simulink model "float_mch_LocalMaxima_HardThreshold"  (R2020a)
settings: Solver=VariableStepAuto  StartTime=0.0  StopTime=10  RelTol=1e-3
model workspace (MAT data in the model file):
  a = 0
values from neighbouring files (symbols this model uses):
  fs = 30000    [float_mch_run_LocalMaxima_AdaptiveThreshold.m]    (also in float_mch_run_LocalMaxima_HardThreshold.m)
libraries: dspfdesign x2, dspswit3 x1, simulink x1
settings Model: SimulationMode=accelerator  Creator=sbuccelli  LastModifiedBy=diflo

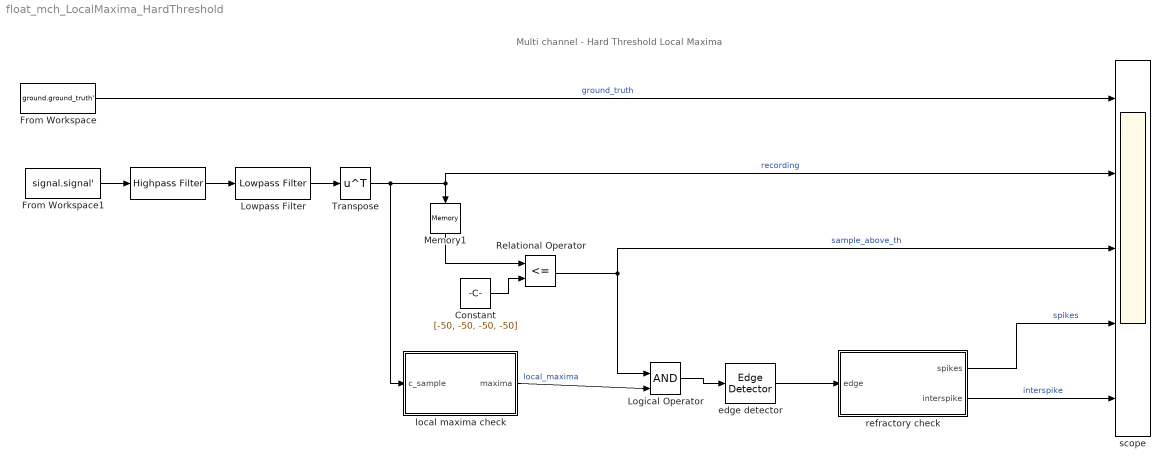
== system float_mch_LocalMaxima_HardThreshold ==
  note: Multi channel - Hard Threshold Local Maxima
  " " : dspfdesign/Highpass Filter  FilterType=IIR  DesignForMinimumOrder=on  FilterOrder=50  StopbandFrequency=1  PassbandFrequency=300  StopbandAttenuation=80  PassbandRipple=0.1  InheritSampleRate=off  SampleRate=30000  SimulateUsing=Interpreted execution  roundingMode=Floor  coeffsDataTypeStr=fixdt(1,16)
  Constant : Constant  Value=[-50, -50, -50, -50]
  From Workspace : FromWorkspace  VariableName=ground.ground_truth'  SampleTime=1/fs
  From Workspace1 : FromWorkspace  VariableName=signal.signal'  SampleTime=1/fs
  Logical Operator : Logic  IconShape=distinctive  AllPortsSameDT=off  OutDataTypeStr=boolean
  Lowpass Filter : dspfdesign/Lowpass Filter  FilterType=IIR  DesignForMinimumOrder=on  FilterOrder=3  PassbandFrequency=3500  StopbandFrequency=8500  PassbandRipple=0.1  StopbandAttenuation=80  InheritSampleRate=off  SampleRate=30000  SimulateUsing=Interpreted execution  roundingMode=Floor  coeffsDataTypeStr=fixdt(1,16)
  Memory1 : Memory  InheritSampleTime=on
  Relational Operator : RelationalOperator  Operator=<=  OutDataTypeStr=boolean  RndMeth=Simplest
  Transpose : Math  Operator=transpose  SaturateOnIntegerOverflow=on
  edge detector : dspswit3/Edge Detector  InputProcessing=Columns as channels (frame based)
      settings: SourceProductBaseCode=DS
  local maxima check : Subsystem
  refractory check : Subsystem
  scope : Scope  NumInputPorts=5
  wires:
  refractory check/1(spikes) -> scope/4  "spikes"
  refractory check/2(interspike) -> scope/5  "interspike"
  From Workspace/1 -> scope/1  "ground_truth"
  edge detector/1 -> refractory check/1("edge  ")
  Relational Operator/1 -> scope/3, Logical Operator/1  "sample_above_th"
  Logical Operator/1 -> edge detector/1
  local maxima check/1(maxima) -> Logical Operator/2  "local_maxima"
  Memory1/1 -> Relational Operator/1
  From Workspace1/1 -> " "/1
  Constant/1 -> Relational Operator/2
  " "/1 -> Lowpass Filter/1
  Lowpass Filter/1 -> Transpose/1
  Transpose/1 -> local maxima check/1(c_sample), scope/2, Memory1/1  "recording"

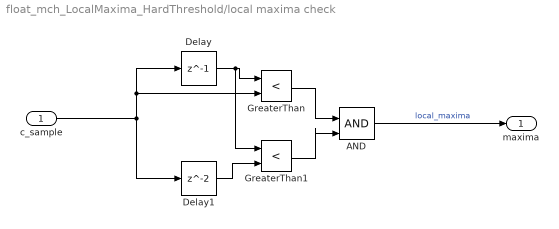
== system float_mch_LocalMaxima_HardThreshold/local maxima check ==
  c_sample : Inport
  AND : Logic  IconShape=distinctive  AllPortsSameDT=off  OutDataTypeStr=boolean
  Delay : Delay  DelayLength=1  SampleTime=1/30000
  Delay1 : Delay  SampleTime=1/30000
  GreaterThan : RelationalOperator  Operator=<  OutDataTypeStr=boolean  RndMeth=Simplest
  GreaterThan1 : RelationalOperator  Operator=<  OutDataTypeStr=boolean  RndMeth=Simplest
  maxima : Outport
  wires:
  Delay/1 -> GreaterThan1/1, GreaterThan/1
  c_sample/1 -> Delay/1, GreaterThan/2, Delay1/1
  GreaterThan/1 -> AND/1
  GreaterThan1/1 -> AND/2
  AND/1 -> maxima/1  "local_maxima"
  Delay1/1 -> GreaterThan1/2

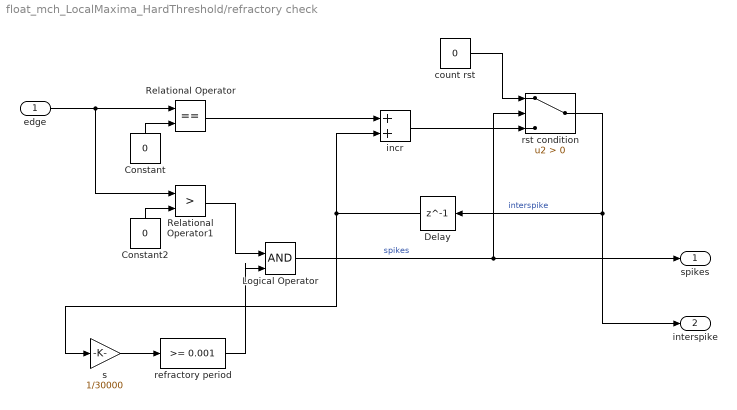
== system float_mch_LocalMaxima_HardThreshold/refractory check ==
  "edge  " : Inport
  Constant : Constant  Value=0
  Constant2 : Constant  Value=0
  Delay : Delay  DelayLength=1  InitialCondition=1
  Logical Operator : Logic  IconShape=distinctive  AllPortsSameDT=off  OutDataTypeStr=boolean
  Relational Operator : RelationalOperator  Operator===  OutDataTypeStr=boolean  RndMeth=Simplest
  Relational Operator1 : RelationalOperator  Operator=>  OutDataTypeStr=boolean  RndMeth=Simplest
  count rst : Constant  Value=0
  incr : Sum  AccumDataTypeStr=double
  refractory period : simulink/Logic and Bit Operations/Compare To Constant  relop=>=  const=0.001  OutDataTypeStr=boolean
  rst condition : Switch  Criteria=u2 > Threshold  OutDataTypeStr=double
  s : Gain  Gain=1/30000
  spikes : Outport
  interspike : Outport  Port=2
  wires:
  count rst/1 -> rst condition/1
  Constant/1 -> Relational Operator/2
  Constant2/1 -> Relational Operator1/2
  Relational Operator1/1 -> Logical Operator/1
  refractory period/1 -> Logical Operator/2
  Logical Operator/1 -> spikes/1, rst condition/2  "spikes"
  incr/1 -> rst condition/3
  rst condition/1 -> interspike/1, Delay/1  "interspike"
  Delay/1 -> s/1, incr/2
  Relational Operator/1 -> incr/1
  "edge  "/1 -> Relational Operator1/1, Relational Operator/1
  s/1 -> refractory period/1
